simulink model "Ex2"  (R2021a)
settings: Solver=VariableStepAuto  StartTime=0.0  StopTime=10.0  RelTol=1e-3
undefined symbols (not defined in the file): c, m
settings Model: Creator=eduma  LastModifiedBy=eduma

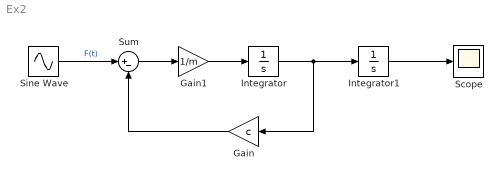
== system Ex2 ==
  Gain : Gain  Gain=c
  Gain1 : Gain  Gain=1/m
  Integrator : Integrator
  Integrator1 : Integrator
  Scope : Scope
  Sine Wave : Sin  Frequency=10*pi  SampleTime=0
  Sum : Sum  Inputs=|+-
  wires:
  Integrator/1 -> Gain/1, Integrator1/1
  Sum/1 -> Gain1/1
  Gain1/1 -> Integrator/1
  Gain/1 -> Sum/2
  Sine Wave/1 -> Sum/1  "F(t)"
  Integrator1/1 -> Scope/1
